simulink model "aprox_delta_dirac"  (R2021a)
settings: Solver=VariableStepAuto  StartTime=0.999  StopTime=1.01  MaxStep=0.000001  RelTol=1e-5
settings Model: Creator=Bremdows  LastModifiedBy=Bremdows

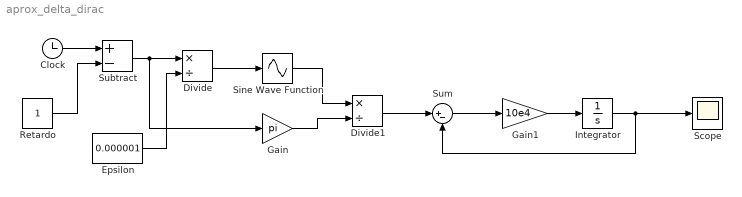
== system aprox_delta_dirac ==
  Clock : Clock
  Divide : Product  Inputs=*/
  Divide1 : Product  Inputs=*/
  Epsilon : Constant  Value=0.000001
  Gain : Gain  Gain=pi
  Gain1 : Gain  Gain=10e4
  Integrator : Integrator
  Retardo : Constant
  Scope : Scope
  Sine Wave Function : Sin  TimeSource=Use external signal  SampleTime=0
  Subtract : Sum  Inputs=+-
  Sum : Sum  Inputs=|+-
  wires:
  Clock/1 -> Subtract/1
  Retardo/1 -> Subtract/2
  Subtract/1 -> Gain/1, Divide/1
  Epsilon/1 -> Divide/2
  Divide/1 -> Sine Wave Function/1
  Gain/1 -> Divide1/2
  Sine Wave Function/1 -> Divide1/1
  Divide1/1 -> Sum/1
  Sum/1 -> Gain1/1
  Gain1/1 -> Integrator/1
  Integrator/1 -> Scope/1, Sum/2
